simulink model "PathFollowing_and_EstimationPosition"  (R2019a)
settings: Solver=VariableStepAuto  StartTime=0.0  StopTime=10.0  RelTol=1e-3
values from neighbouring files (symbols this model uses):
  kx = 10    [Pathfollowing_simulation.m]
  ky = 25    [Pathfollowing_simulation.m]
undefined symbols (not defined in the file or in its folder): kt
libraries: simulink x4
settings Model: Creator=robot  LastModifiedBy=robot

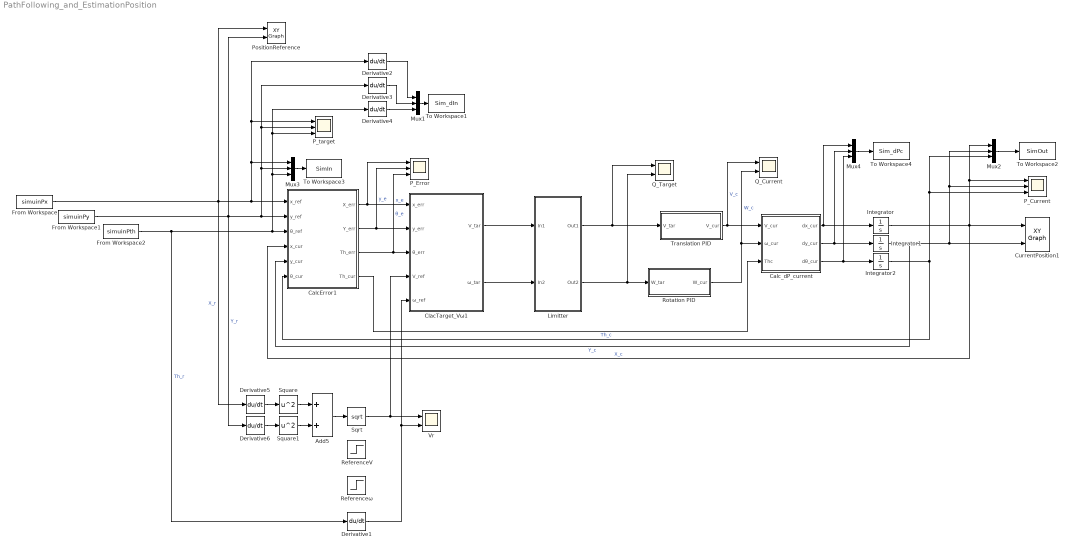
== system PathFollowing_and_EstimationPosition ==
  Add5 : Sum
  CalcError1 : Subsystem  TreatAsAtomicUnit=on
      settings: RTWSystemCode=Nonreusable function
  Calc_dP_current : Subsystem
  ClacTarget_Vω1 : Subsystem
  CurrentPosition1 : simulink/Sinks/XY Graph  xmin=-200  xmax=200  ymin=-10  ymax=400  st=-1
  Derivative{1..6} (6 alike) : Derivative
  From Workspace : FromWorkspace  VariableName=simuinPx  SampleTime=0
  From Workspace1 : FromWorkspace  VariableName=simuinPy  SampleTime=0
  From Workspace2 : FromWorkspace  VariableName=simuinPth  SampleTime=0
  Integrator : Integrator
  Integrator1 : Integrator
  Integrator2 : Integrator
  Limitter : Subsystem
  Mux{1..4} (4 alike) : Mux  Inputs=3
  P_Current : Scope  NumInputPorts=3
  P_Error : Scope  NumInputPorts=3
  P_target : Scope  NumInputPorts=3
  PositionReference : simulink/Sinks/XY Graph  xmin=-200  xmax=200  ymin=-10  ymax=400  st=-1
  Q_Current : Scope  NumInputPorts=2
  Q_Target : Scope  NumInputPorts=2
  ReferenceV : Step  Time=0  After=65  SampleTime=0.001
  Referenceω : Step  Time=0  After=0  SampleTime=0.001
  Rotation PID : Subsystem
  Sqrt : Sqrt  SaturateOnIntegerOverflow=on
  Square : Math  Operator=square  SaturateOnIntegerOverflow=on
  Square1 : Math  Operator=square  SaturateOnIntegerOverflow=on
  To Workspace1 : ToWorkspace  VariableName=Sim_dIn  SampleTime=-1
  To Workspace2 : ToWorkspace  VariableName=SimOut  SampleTime=-1
  To Workspace3 : ToWorkspace  VariableName=SimIn  SampleTime=-1
  To Workspace4 : ToWorkspace  VariableName=Sim_dPc  SampleTime=-1
  Translation PID : Subsystem  TreatAsAtomicUnit=on
  Vr : Scope  NumInputPorts=2
  wires:
  Limitter/1(Out1) -> Q_Target/1, Translation PID/1(V_tar)
  Derivative5/1 -> Square/1
  Translation PID/1(V_cur) -> Q_Current/1, Calc_dP_current/1(V_cur)  "V_c"
  ClacTarget_Vω1/1(V_tar) -> Limitter/1(In1)
  Limitter/2(Out2) -> Q_Target/2, Rotation PID/1(W_tar)
  From Workspace1/1 -> Derivative6/1, CalcError1/2(y_ref), Derivative3/1, P_target/2, Mux3/2, PositionReference/2  "Y_r"
  Derivative3/1 -> Mux1/2
  ClacTarget_Vω1/2(ω_tar) -> Limitter/2(In2)
  Derivative1/1 -> Vr/2, ClacTarget_Vω1/5(ω_ref)
  Integrator1/1 -> Mux2/2, P_Current/2, CurrentPosition1/2, CalcError1/5(y_cur)  "Y_c"
  Derivative2/1 -> Mux1/1
  Rotation PID/1(W_cur) -> Q_Current/2, Calc_dP_current/2(ω_cur)  "W_c"
  Square1/1 -> Add5/2
  Calc_dP_current/3(dθ_cur) -> Mux4/3, Integrator2/1
  CalcError1/3(Th_err) -> P_Error/3, ClacTarget_Vω1/3(θ_err)  "θ_e"
  Mux4/1 -> To Workspace4/1
  Calc_dP_current/1(dx_cur) -> Mux4/1, Integrator/1
  From Workspace2/1 -> CalcError1/3(θ_ref), Derivative4/1, P_target/3, Mux3/3, Derivative1/1  "Th_r"
  CalcError1/4(Th_cur) -> Calc_dP_current/3(Thc)
  Derivative4/1 -> Mux1/3
  Mux2/1 -> To Workspace2/1
  Mux1/1 -> To Workspace1/1
  CalcError1/2(Y_err) -> P_Error/2, ClacTarget_Vω1/2(y_err)  "y_e"
  From Workspace/1 -> Derivative5/1, PositionReference/1, CalcError1/1(x_ref), P_target/1, Derivative2/1, Mux3/1  "X_r"
  CalcError1/1(X_err) -> P_Error/1, ClacTarget_Vω1/1(x_err)  "x_e"
  Square/1 -> Add5/1
  Add5/1 -> Sqrt/1
  Mux3/1 -> To Workspace3/1
  Calc_dP_current/2(dy_cur) -> Mux4/2, Integrator1/1
  Integrator/1 -> Mux2/1, P_Current/1, CurrentPosition1/1, CalcError1/4(x_cur)  "X_c"
  Derivative6/1 -> Square1/1
  Integrator2/1 -> Mux2/3, P_Current/3, CalcError1/6(θ_cur)  "Th_c"
  Sqrt/1 -> Vr/1, ClacTarget_Vω1/4(V_ref)

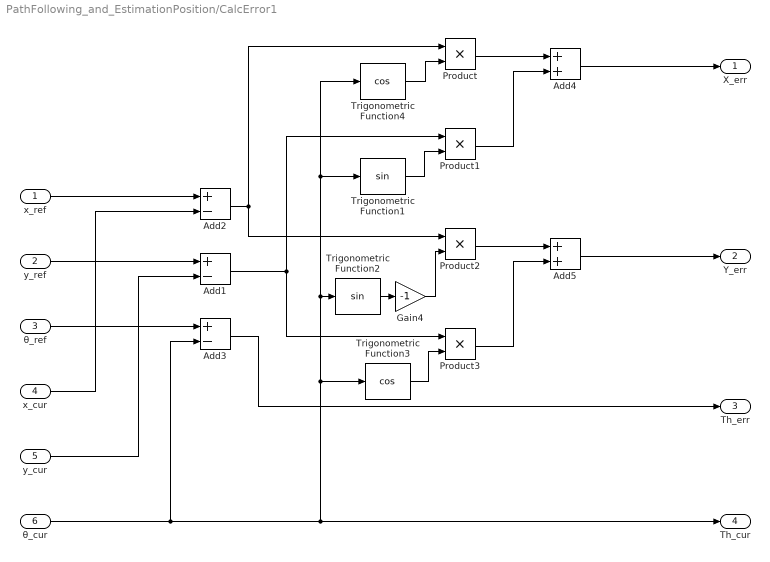
== system PathFollowing_and_EstimationPosition/CalcError1 ==
  x_ref : Inport
  y_ref : Inport  Port=2
  θ_ref : Inport  Port=3
  x_cur : Inport  Port=4
  y_cur : Inport  Port=5
  θ_cur : Inport  Port=6
  Add1 : Sum  Inputs=+-
  Add2 : Sum  Inputs=+-
  Add3 : Sum  Inputs=+-
  Add4 : Sum
  Add5 : Sum
  Gain4 : Gain  Gain=-1
  Product{,1..3} (4 alike) : Product
  Trigonometric Function1 : Trigonometry
  Trigonometric Function2 : Trigonometry
  Trigonometric Function3 : Trigonometry  Operator=cos
  Trigonometric Function4 : Trigonometry  Operator=cos
  X_err : Outport
  Y_err : Outport  Port=2
  Th_err : Outport  Port=3
  Th_cur : Outport  Port=4
  wires:
  x_cur/1 -> Add2/2
  x_ref/1 -> Add2/1
  y_ref/1 -> Add1/1
  y_cur/1 -> Add1/2
  θ_cur/1 -> Th_cur/1, Trigonometric Function4/1, Trigonometric Function1/1, Trigonometric Function2/1, Trigonometric Function3/1, Add3/2
  Trigonometric Function4/1 -> Product/2
  Product/1 -> Add4/1
  Trigonometric Function1/1 -> Product1/2
  Add1/1 -> Product3/1, Product1/1
  Product1/1 -> Add4/2
  Add4/1 -> X_err/1
  Add3/1 -> Th_err/1
  Add2/1 -> Product2/1, Product/1
  Product2/1 -> Add5/1
  Trigonometric Function3/1 -> Product3/2
  Product3/1 -> Add5/2
  Add5/1 -> Y_err/1
  Trigonometric Function2/1 -> Gain4/1
  Gain4/1 -> Product2/2
  θ_ref/1 -> Add3/1

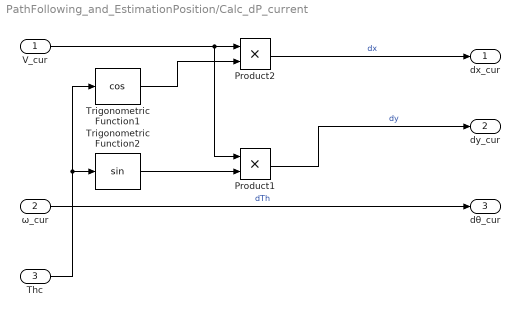
== system PathFollowing_and_EstimationPosition/Calc_dP_current ==
  V_cur : Inport
  ω_cur : Inport  Port=2
  Thc : Inport  Port=3
  Product1 : Product
  Product2 : Product
  Trigonometric Function1 : Trigonometry  Operator=cos
  Trigonometric Function2 : Trigonometry
  dx_cur : Outport
  dy_cur : Outport  Port=2
  dθ_cur : Outport  Port=3
  wires:
  V_cur/1 -> Product2/1, Product1/1
  Trigonometric Function1/1 -> Product2/2
  Thc/1 -> Trigonometric Function2/1, Trigonometric Function1/1
  Product2/1 -> dx_cur/1  "dx"
  Product1/1 -> dy_cur/1  "dy"
  Trigonometric Function2/1 -> Product1/2
  ω_cur/1 -> dθ_cur/1  "dTh"

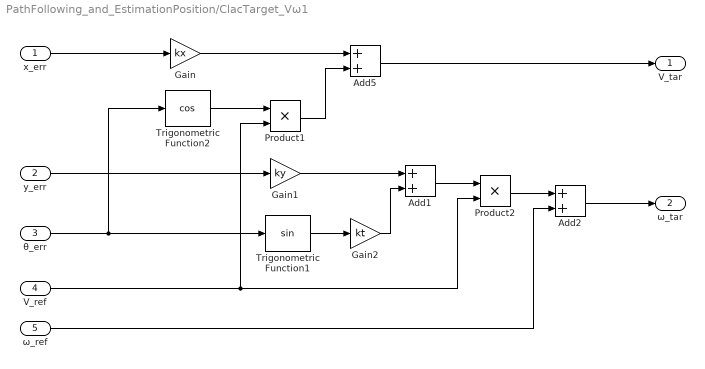
== system PathFollowing_and_EstimationPosition/ClacTarget_Vω1 ==
  x_err : Inport
  y_err : Inport  Port=2
  θ_err : Inport  Port=3
  V_ref : Inport  Port=4
  ω_ref : Inport  Port=5
  Add1 : Sum
  Add2 : Sum
  Add5 : Sum
  Gain : Gain  Gain=kx
  Gain1 : Gain  Gain=ky
  Gain2 : Gain  Gain=kt
  Product1 : Product
  Product2 : Product
  Trigonometric Function1 : Trigonometry
  Trigonometric Function2 : Trigonometry  Operator=cos
  V_tar : Outport
  ω_tar : Outport  Port=2
  wires:
  x_err/1 -> Gain/1
  Gain/1 -> Add5/1
  θ_err/1 -> Trigonometric Function1/1, Trigonometric Function2/1
  Trigonometric Function2/1 -> Product1/1
  V_ref/1 -> Product2/2, Product1/2
  Product1/1 -> Add5/2
  Add5/1 -> V_tar/1
  y_err/1 -> Gain1/1
  Gain1/1 -> Add1/1
  Trigonometric Function1/1 -> Gain2/1
  Gain2/1 -> Add1/2
  Add1/1 -> Product2/1
  Product2/1 -> Add2/1
  ω_ref/1 -> Add2/2
  Add2/1 -> ω_tar/1

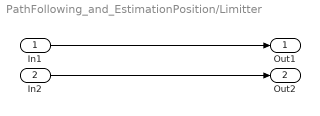
== system PathFollowing_and_EstimationPosition/Limitter ==
  In1 : Inport
  In2 : Inport  Port=2
  Out1 : Outport
  Out2 : Outport  Port=2
  wires:
  In1/1 -> Out1/1
  In2/1 -> Out2/1

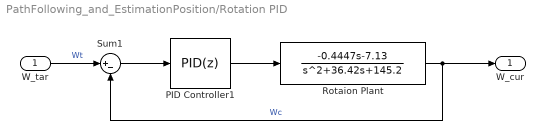
== system PathFollowing_and_EstimationPosition/Rotation PID ==
  W_tar : Inport
  PID Controller1 : simulink/Continuous/PID Controller  Controller=PID  Form=Parallel  TimeDomain=Discrete-time  SampleTime=0.001  IntegratorMethod=Forward Euler  FilterMethod=Forward Euler  ControllerParametersSource=internal  P=-218.8515  I=-4309.9877  D=0  UseFilter=on  N=100  TunerSelectOption=Transfer Function Based (PID Tuner App)  InitialConditionSource=internal  InitialConditionForIntegrator=0  InitialConditionForFilter=0  DifferentiatorICPrevScaledInput=0  ExternalReset=none  TrackingMode=off  Kt=1  LimitOutput=on  UpperSaturationLimit=1200  LowerSaturationLimit=-1200  LinearizeAsGain=on  AntiWindupMode=none  Kb=1  POutMin=[]  POutMax=[]  IOutMin=[]  IOutMax=[]  DOutMin=[]  DOutMax=[]  NOutMin=[]  NOutMax=[]  SumOutMin=[]  SumOutMax=[]  SaturationOutMin=[]  SaturationOutMax=[]  PParamMin=[]  PParamMax=[]  IParamMin=[]  IParamMax=[]  DParamMin=[]  DParamMax=[]  NParamMin=[]  NParamMax=[]  KbParamMin=[]  KbParamMax=[]  KtParamMin=[]  KtParamMax=[]  KbOutMin=[]  KbOutMax=[]  KtOutMin=[]  KtOutMax=[]  IntegratorOutMin=[]  IntegratorOutMax=[]  FilterOutMin=[]  FilterOutMax=[]  SumI1OutMin=[]  SumI1OutMax=[]  SumI2OutMin=[]  SumI2OutMax=[]  SumI3OutMin=[]  SumI3OutMax=[]  SumI4OutMin=[]  SumI4OutMax=[]  SumDOutMin=[]  SumDOutMax=[]  DifferentiatorOutMin=[]  DifferentiatorOutMax=[]  FilterDiffOutCoefMin=[]  FilterDiffOutCoefMax=[]  ReciprocalOutMin=[]  ReciprocalOutMax=[]  SumDenOutMin=[]  SumDenOutMax=[]  SumNumOutMin=[]  SumNumOutMax=[]  DivideOutMin=[]  DivideOutMax=[]  IntegratorContinuousStateAttributes=''  IntegratorStateMustResolveToSignalObject=off  IntegratorRTWStateStorageClass=Auto  FilterContinuousStateAttributes=''  FilterStateMustResolveToSignalObject=off  FilterRTWStateStorageClass=Auto  ParallelPVariant=InternalParameters  IdealPVariant=Disabled  IVariant=InternalParameters  DVariant=InternalParameters  IntegratorVariant=Discrete  SatVariant=Enabled  AWVariant=Passthrough  PCopyVariant=Disabled  TRVariant=Disabled  FdbkBlocksVariant=Forward  IdealPFdbkVariant=Disabled  SatFdbkVariant=Disabled  DerivativeFilterVariant=ForwardEulerFilter  NVariant=InternalParameters  NCopyVariant=Disabled  FilterICVariant=InternalICsFilter  IntegratorICVariant=InternalICs  ExternalResetVariant=Disabled  TRSumVariant=Passthrough  SumFdbkVariant=Disabled  SumVariant=Sum_PID
  Rotaion Plant : TransferFcn  Numerator=[-0.4447 -7.13]  Denominator=[1 36.42 145.2]
  Sum1 : Sum  Inputs=|+-
  W_cur : Outport
  wires:
  PID Controller1/1 -> Rotaion Plant/1
  Sum1/1 -> PID Controller1/1
  W_tar/1 -> Sum1/1  "Wt"
  Rotaion Plant/1 -> Sum1/2, W_cur/1  "Wc"

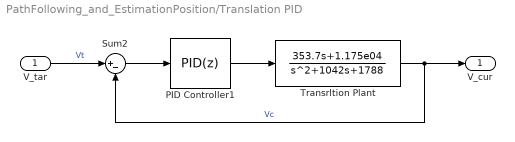
== system PathFollowing_and_EstimationPosition/Translation PID ==
  V_tar : Inport
  PID Controller1 : simulink/Continuous/PID Controller  Controller=PID  Form=Parallel  TimeDomain=Discrete-time  SampleTime=0.001  IntegratorMethod=Forward Euler  FilterMethod=Forward Euler  ControllerParametersSource=internal  P=0.73598  I=3.7518  D=0  UseFilter=on  N=100  TunerSelectOption=Transfer Function Based (PID Tuner App)  InitialConditionSource=internal  InitialConditionForIntegrator=0  InitialConditionForFilter=0  DifferentiatorICPrevScaledInput=0  ExternalReset=none  TrackingMode=off  Kt=1  LimitOutput=on  UpperSaturationLimit=1200  LowerSaturationLimit=-1200  LinearizeAsGain=on  AntiWindupMode=none  Kb=1  POutMin=[]  POutMax=[]  IOutMin=[]  IOutMax=[]  DOutMin=[]  DOutMax=[]  NOutMin=[]  NOutMax=[]  SumOutMin=[]  SumOutMax=[]  SaturationOutMin=[]  SaturationOutMax=[]  PParamMin=[]  PParamMax=[]  IParamMin=[]  IParamMax=[]  DParamMin=[]  DParamMax=[]  NParamMin=[]  NParamMax=[]  KbParamMin=[]  KbParamMax=[]  KtParamMin=[]  KtParamMax=[]  KbOutMin=[]  KbOutMax=[]  KtOutMin=[]  KtOutMax=[]  IntegratorOutMin=[]  IntegratorOutMax=[]  FilterOutMin=[]  FilterOutMax=[]  SumI1OutMin=[]  SumI1OutMax=[]  SumI2OutMin=[]  SumI2OutMax=[]  SumI3OutMin=[]  SumI3OutMax=[]  SumI4OutMin=[]  SumI4OutMax=[]  SumDOutMin=[]  SumDOutMax=[]  DifferentiatorOutMin=[]  DifferentiatorOutMax=[]  FilterDiffOutCoefMin=[]  FilterDiffOutCoefMax=[]  ReciprocalOutMin=[]  ReciprocalOutMax=[]  SumDenOutMin=[]  SumDenOutMax=[]  SumNumOutMin=[]  SumNumOutMax=[]  DivideOutMin=[]  DivideOutMax=[]  IntegratorContinuousStateAttributes=''  IntegratorStateMustResolveToSignalObject=off  IntegratorRTWStateStorageClass=Auto  FilterContinuousStateAttributes=''  FilterStateMustResolveToSignalObject=off  FilterRTWStateStorageClass=Auto  ParallelPVariant=InternalParameters  IdealPVariant=Disabled  IVariant=InternalParameters  DVariant=InternalParameters  IntegratorVariant=Discrete  SatVariant=Enabled  AWVariant=Passthrough  PCopyVariant=Disabled  TRVariant=Disabled  FdbkBlocksVariant=Forward  IdealPFdbkVariant=Disabled  SatFdbkVariant=Disabled  DerivativeFilterVariant=ForwardEulerFilter  NVariant=InternalParameters  NCopyVariant=Disabled  FilterICVariant=InternalICsFilter  IntegratorICVariant=InternalICs  ExternalResetVariant=Disabled  TRSumVariant=Passthrough  SumFdbkVariant=Disabled  SumVariant=Sum_PID
  Sum2 : Sum  Inputs=|+-
  Transrltion Plant : TransferFcn  Numerator=[353.7 1.175e04]  Denominator=[1 1042 1788]
  V_cur : Outport
  wires:
  Sum2/1 -> PID Controller1/1
  PID Controller1/1 -> Transrltion Plant/1
  Transrltion Plant/1 -> V_cur/1, Sum2/2  "Vc"
  V_tar/1 -> Sum2/1  "Vt"
